simulink model "nms3D_2021"  (R2021a)
settings: Solver=ode15s  StartTime=0.0  StopTime=2  MaxStep=1e-2  RelTol=1e-2
StartFcn:
  | tic
StopFcn:
  | toc
  | 
  | 
  | %if GimbalLockFlag
  |  % fprintf(2, 'Almost reached Gimbal Lock of IMU. Simulation stopped.\n')
  | %end
  | 
  | %fprintf('Elapsed time: %4.2f sec (%4.2f%% realtime)\n', a, tout(end)/a*100)
values from neighbouring files (symbols this model uses):
  Balance02 = pMod(24:29)    [AssignSimulinkParams.m]    (also in assign_parameters.m = param(26:29))
  Balance13 = pMod(30:35)    [AssignSimulinkParams.m]    (also in assign_parameters.m = param(30:33))
  BalanceTrunk = pMod(22:23)    [AssignSimulinkParams.m]    (also in assign_parameters.m = param(22:23))
  BalanceTrunkLat = param(24:25)    [assign_parameters.m]
  BalanceTrunkLatOld = pMod(43:46)    [AssignSimulinkParams.m]    (also in assign_parameters.m = param(43:46))
  BalanceTrunkOld = param(49:53)    [assign_parameters.m]
  BasisStim = pMod(1:11)    [AssignSimulinkParams.m]    (also in assign_parameters.m = param(1:11))
  CompliantLeg = pMod(12:14)    [AssignSimulinkParams.m]    (also in assign_parameters.m = param(12:14))
  CompliantLegLat = pMod(15)    [AssignSimulinkParams.m]    (also in assign_parameters.m = param(15))
  PreventKneeOverextension = pMod(16:21)    [AssignSimulinkParams.m]    (also in assign_parameters.m = param(16:21))
  SwingCompLatOld = param(47:48)    [assign_parameters.m]
  Target02 = pMod(36:38)    [AssignSimulinkParams.m]    (also in assign_parameters.m = param(34:36))
  Target02_va = pMod(49:54)    [AssignSimulinkParams.m]    (also in assign_parameters.m = param(60:65))
  Target13 = pMod(39:41)    [AssignSimulinkParams.m]    (also in assign_parameters.m = param(37:39))
  Target13_va = pMod(55:60)    [AssignSimulinkParams.m]    (also in assign_parameters.m = param(66:71))
  theta0_world = param(59)    [assign_parameters.m]
  WramameiSL_1000 = readmatrix('WSL_1000_Norm_Sigmoid_MSE_cont.csv')    [nms3D_prep.m]
  ZramameiSL_1000 = readmatrix('ZSL_1000_Norm_Sigmoid_MSE_cont.csv')    [nms3D_prep.m]
undefined symbols (not defined in the file or in its folder): ICs, mParams, X, Y, Z
libraries: nesl_utility x106, sm_lib x87, simulink x70, eeGeneralControl x28, robotmaniplib x14, dspinverses x10, robotcorelib x5, dspmathops x3, vrlib x1, pid_lib x1
(part 2 of 8)

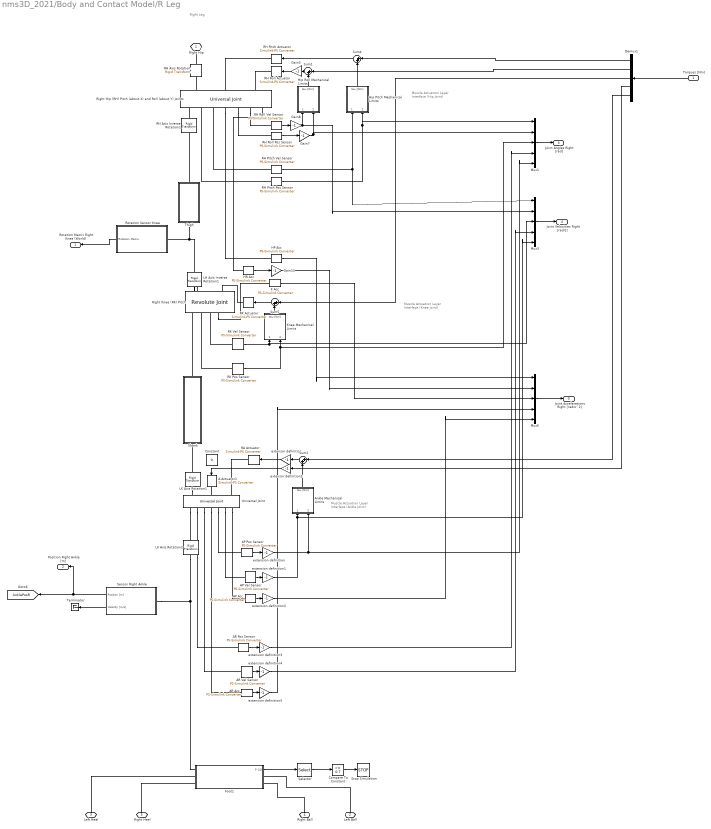
== system nms3D_2021/Body and Contact Model/R Leg ==
  note: Muscle Actuation
      | Layer Interface
      | (Hip Joint)
  note: Muscle Actuation
      | Layer Interface
      | (Knee Joint)
  note: Muscle Actuation
      | Layer Interface
      | (Ankle Joint)
  note: Right Leg
  Torques [Nm] : Inport
  A Actuator1 : nesl_utility/Simulink-PS Converter  PhysicalDomain=network_engine_domain  SubClassName=ps_input  LeftPortType=input  RightPortType=output  PseudoPeriodic=off  Frequencies=[]  NoiseDistribution=none  NoiseParameters=[]  Unit=N*m  AffineConversion=off  FilteringAndDerivatives=zero  SimscapeFilterOrder=1  InputFilterTimeConstant=.001  UdotUserProvided=0
      settings: SourceProductBaseCode=PW,SS
  AP Acc : nesl_utility/PS-Simulink Converter  PhysicalDomain=network_engine_domain  SubClassName=ps_output  LeftPortType=input  RightPortType=output  PseudoPeriodic=off  Frequencies=[]  Unit=rad/(s^2)  AffineConversion=off
      settings: SourceProductBaseCode=PW,SS
  AP Pos Sensor : nesl_utility/PS-Simulink Converter  PhysicalDomain=network_engine_domain  SubClassName=ps_output  LeftPortType=input  RightPortType=output  PseudoPeriodic=off  Frequencies=[]  Unit=rad  AffineConversion=off
      settings: SourceProductBaseCode=PW,SS
  AP Vel Sensor : nesl_utility/PS-Simulink Converter  PhysicalDomain=network_engine_domain  SubClassName=ps_output  LeftPortType=input  RightPortType=output  PseudoPeriodic=off  Frequencies=[]  Unit=rad/s  AffineConversion=off
      settings: SourceProductBaseCode=PW,SS
  AR Acc : nesl_utility/PS-Simulink Converter  PhysicalDomain=network_engine_domain  SubClassName=ps_output  LeftPortType=input  RightPortType=output  PseudoPeriodic=off  Frequencies=[]  Unit=rad/(s^2)  AffineConversion=off
      settings: SourceProductBaseCode=PW,SS
  AR Pos Sensor : nesl_utility/PS-Simulink Converter  PhysicalDomain=network_engine_domain  SubClassName=ps_output  LeftPortType=input  RightPortType=output  PseudoPeriodic=off  Frequencies=[]  Unit=rad  AffineConversion=off
      settings: SourceProductBaseCode=PW,SS
  AR Vel Sensor : nesl_utility/PS-Simulink Converter  PhysicalDomain=network_engine_domain  SubClassName=ps_output  LeftPortType=input  RightPortType=output  PseudoPeriodic=off  Frequencies=[]  Unit=rad/s  AffineConversion=off
      settings: SourceProductBaseCode=PW,SS
  Ankle Mechanical Limits : Subsystem
  Compare To Constant : simulink/Logic and Bit Operations/Compare To Constant  relop=>=  const=0.7  OutDataTypeStr=boolean
  Constant : Constant  Value=0
  Demux1 : Demux  Outputs=5
  Foot1 : Subsystem
  Gain{3,7..8,11} (4 alike) : Gain  Gain=-1
  HP Acc : nesl_utility/PS-Simulink Converter  PhysicalDomain=network_engine_domain  SubClassName=ps_output  LeftPortType=input  RightPortType=output  PseudoPeriodic=off  Frequencies=[]  Unit=rad/(s^2)  AffineConversion=off
      settings: SourceProductBaseCode=PW,SS
  HR Acc : nesl_utility/PS-Simulink Converter  PhysicalDomain=network_engine_domain  SubClassName=ps_output  LeftPortType=input  RightPortType=output  PseudoPeriodic=off  Frequencies=[]  Unit=rad/(s^2)  AffineConversion=off
      settings: SourceProductBaseCode=PW,SS
  Hip Pitch Mechanical Limits : Subsystem
  Hip Roll Mechanical Limits : Subsystem
  K Acc : nesl_utility/PS-Simulink Converter  PhysicalDomain=network_engine_domain  SubClassName=ps_output  LeftPortType=input  RightPortType=output  PseudoPeriodic=off  Frequencies=[]  Unit=rad/(s^2)  AffineConversion=off
      settings: SourceProductBaseCode=PW,SS
  Knee Mechanical Limits : Subsystem
  LH Axis Inverse Rotation1 : sm_lib/Frames and Transforms/Rigid Transform  TranslationMethod=None  TranslationStandardOffset=-0.5  TranslationLengthUnit=m  TranslationStandardAxis=+Y  TranslationCartesianOffset=0  TranslationROffset=0  TranslationROffsetUnits=m  TranslationZOffset=0  TranslationZOffsetUnits=m  TranslationThetaOffset=0  TranslationThetaOffsetUnits=deg  RotationMethod=RotationSequence  RotationAngleUnits=deg  RotationStandardAxis=+X  RotationAngle=-90  RotationArbitraryAxis=[0 0 1]  FollAlignAxisA=+X  BaseAlignAxisA=+Y  FollAlignAxisB=+Y  BaseAlignAxisB=+Z  RotationSequenceAxes=BaseAxes  RotationSequence=ZXZ  RotationSequenceAngles=[180 0 0]  RotationSequenceAnglesUnits=deg  RotationMatrix=[1 0 0; 0 1 0; 0 0 1]
  LK Axis Rotation1 : sm_lib/Frames and Transforms/Rigid Transform  TranslationMethod=None  TranslationStandardOffset=-0.5  TranslationLengthUnit=m  TranslationStandardAxis=+Y  TranslationCartesianOffset=0  TranslationROffset=0  TranslationROffsetUnits=m  TranslationZOffset=0  TranslationZOffsetUnits=m  TranslationThetaOffset=0  TranslationThetaOffsetUnits=deg  RotationMethod=StandardAxis  RotationAngleUnits=deg  RotationStandardAxis=+X  RotationAngle=90  RotationArbitraryAxis=[0 0 1]  FollAlignAxisA=+X  BaseAlignAxisA=+Y  FollAlignAxisB=+Y  BaseAlignAxisB=+Z  RotationSequenceAxes=BaseAxes  RotationSequence=ZXZ  RotationSequenceAngles=[180 0 0]  RotationSequenceAnglesUnits=deg  RotationMatrix=[1 0 0; 0 1 0; 0 0 1]
  LK Axis Rotation2 : sm_lib/Frames and Transforms/Rigid Transform  TranslationMethod=None  TranslationStandardOffset=-0.5  TranslationLengthUnit=m  TranslationStandardAxis=+Y  TranslationCartesianOffset=0  TranslationROffset=0  TranslationROffsetUnits=m  TranslationZOffset=0  TranslationZOffsetUnits=m  TranslationThetaOffset=0  TranslationThetaOffsetUnits=deg  RotationMethod=StandardAxis  RotationAngleUnits=deg  RotationStandardAxis=+X  RotationAngle=-90  RotationArbitraryAxis=[0 0 1]  FollAlignAxisA=+X  BaseAlignAxisA=+Y  FollAlignAxisB=+Y  BaseAlignAxisB=+Z  RotationSequenceAxes=BaseAxes  RotationSequence=ZXZ  RotationSequenceAngles=[180 0 0]  RotationSequenceAnglesUnits=deg  RotationMatrix=[1 0 0; 0 1 0; 0 0 1]
  Mux1 : Mux  Inputs=5
  Mux3 : Mux  Inputs=5
  Mux5 : Mux  Inputs=5
  RA Actuator : nesl_utility/Simulink-PS Converter  PhysicalDomain=network_engine_domain  SubClassName=ps_input  LeftPortType=input  RightPortType=output  PseudoPeriodic=off  Frequencies=[]  NoiseDistribution=none  NoiseParameters=[]  Unit=N*m  AffineConversion=off  FilteringAndDerivatives=zero  SimscapeFilterOrder=1  InputFilterTimeConstant=.001  UdotUserProvided=0
      settings: SourceProductBaseCode=PW,SS
  RH Pitch Pos Sensor : nesl_utility/PS-Simulink Converter  PhysicalDomain=network_engine_domain  SubClassName=ps_output  LeftPortType=input  RightPortType=output  PseudoPeriodic=off  Frequencies=[]  Unit=rad  AffineConversion=off
      settings: SourceProductBaseCode=PW,SS
  RH Pitch Vel Sensor : nesl_utility/PS-Simulink Converter  PhysicalDomain=network_engine_domain  SubClassName=ps_output  LeftPortType=input  RightPortType=output  PseudoPeriodic=off  Frequencies=[]  Unit=rad/s  AffineConversion=off
      settings: SourceProductBaseCode=PW,SS
  RH Roll Pos Sensor : nesl_utility/PS-Simulink Converter  PhysicalDomain=network_engine_domain  SubClassName=ps_output  LeftPortType=input  RightPortType=output  PseudoPeriodic=off  Frequencies=[]  Unit=rad  AffineConversion=off
      settings: SourceProductBaseCode=PW,SS
  "RH Roll Vel Sensor " : nesl_utility/PS-Simulink Converter  PhysicalDomain=network_engine_domain  SubClassName=ps_output  LeftPortType=input  RightPortType=output  PseudoPeriodic=off  Frequencies=[]  Unit=rad/s  AffineConversion=off
      settings: SourceProductBaseCode=PW,SS
  RH Axis Inverse Rotation1 : sm_lib/Frames and Transforms/Rigid Transform  TranslationMethod=None  TranslationStandardOffset=-0.5  TranslationLengthUnit=m  TranslationStandardAxis=+Y  TranslationCartesianOffset=[0 0.2 0]  TranslationROffset=0  TranslationROffsetUnits=m  TranslationZOffset=0  TranslationZOffsetUnits=m  TranslationThetaOffset=0  TranslationThetaOffsetUnits=deg  RotationMethod=RotationSequence  RotationAngleUnits=deg  RotationStandardAxis=+X  RotationAngle=-90  RotationArbitraryAxis=[0 0 1]  FollAlignAxisA=+X  BaseAlignAxisA=+Y  FollAlignAxisB=+Y  BaseAlignAxisB=+Z  RotationSequenceAxes=BaseAxes  RotationSequence=YXY  RotationSequenceAngles=[ -90 -90 0]  RotationSequenceAnglesUnits=deg  RotationMatrix=[1 0 0; 0 1 0; 0 0 1]
  RH Axis Rotation : sm_lib/Frames and Transforms/Rigid Transform  TranslationMethod=None  TranslationStandardOffset=-0  TranslationLengthUnit=m  TranslationStandardAxis=+Y  TranslationCartesianOffset=0  TranslationROffset=0  TranslationROffsetUnits=m  TranslationZOffset=0  TranslationZOffsetUnits=m  TranslationThetaOffset=0  TranslationThetaOffsetUnits=deg  RotationMethod=RotationSequence  RotationAngleUnits=deg  RotationStandardAxis=+X  RotationAngle=90  RotationArbitraryAxis=[0 0 1]  FollAlignAxisA=+X  BaseAlignAxisA=+Y  FollAlignAxisB=+Y  BaseAlignAxisB=+Z  RotationSequenceAxes=FollowerAxes  RotationSequence=XZX  RotationSequenceAngles=[-90 90 0]  RotationSequenceAnglesUnits=deg  RotationMatrix=[1 0 0; 0 1 0; 0 0 1]
  RH Pitch Actuator : nesl_utility/Simulink-PS Converter  PhysicalDomain=network_engine_domain  SubClassName=ps_input  LeftPortType=input  RightPortType=output  PseudoPeriodic=off  Frequencies=[]  NoiseDistribution=none  NoiseParameters=[]  Unit=N*m  AffineConversion=off  FilteringAndDerivatives=zero  SimscapeFilterOrder=1  InputFilterTimeConstant=.001  UdotUserProvided=0
      settings: SourceProductBaseCode=PW,SS
  RH Roll Actuator : nesl_utility/Simulink-PS Converter  PhysicalDomain=network_engine_domain  SubClassName=ps_input  LeftPortType=input  RightPortType=output  PseudoPeriodic=off  Frequencies=[]  NoiseDistribution=none  NoiseParameters=[]  Unit=N*m  AffineConversion=off  FilteringAndDerivatives=zero  SimscapeFilterOrder=1  InputFilterTimeConstant=.001  UdotUserProvided=0
      settings: SourceProductBaseCode=PW,SS
  RK Actuator : nesl_utility/Simulink-PS Converter  PhysicalDomain=network_engine_domain  SubClassName=ps_input  LeftPortType=input  RightPortType=output  PseudoPeriodic=off  Frequencies=[]  NoiseDistribution=none  NoiseParameters=[]  Unit=N*m  AffineConversion=off  FilteringAndDerivatives=zero  SimscapeFilterOrder=1  InputFilterTimeConstant=.001  UdotUserProvided=0
      settings: SourceProductBaseCode=PW,SS
  RK Pos Sensor : nesl_utility/PS-Simulink Converter  PhysicalDomain=network_engine_domain  SubClassName=ps_output  LeftPortType=input  RightPortType=output  PseudoPeriodic=off  Frequencies=[]  Unit=rad  AffineConversion=off
      settings: SourceProductBaseCode=PW,SS
  RK Vel Sensor : nesl_utility/PS-Simulink Converter  PhysicalDomain=network_engine_domain  SubClassName=ps_output  LeftPortType=input  RightPortType=output  PseudoPeriodic=off  Frequencies=[]  Unit=rad/s  AffineConversion=off
      settings: SourceProductBaseCode=PW,SS
  Right Hip (RH) Pitch (about X) and Roll (about Y) Joints : sm_lib/Joints/Universal Joint  JointMode=Normal  SenseConstraintForce=off  SenseConstraintForceX=off  SenseConstraintForceY=off  SenseConstraintForceZ=off  SenseConstraintTorque=off  SenseConstraintTorqueX=off  SenseConstraintTorqueY=off  SenseConstraintTorqueZ=off  SenseTotalForce=off  SenseTotalForceX=off  SenseTotalForceY=off  SenseTotalForceZ=off  SenseTotalTorque=off  SenseTotalTorqueX=off  SenseTotalTorqueY=off  SenseTotalTorqueZ=off  CompositeWrenchDir=FollowerOnBase  CompositeWrenchFrame=FollowerFrame  RxEquilibriumPosition=0  RxEquilibriumPositionUnits=deg  RxSpringStiffness=0  RxSpringStiffnessUnits=N*m/deg  RxDampingCoefficient=0  RxDampingCoefficientUnits=N*m/(deg/s)  RxTorqueActuationMode=InputTorque  RxMotionActuationMode=ComputedMotion  RxSensePosition=on  RxSenseVelocity=on  RxSenseAcceleration=on  RxSenseTorqueForce=off  RxSenseLowerLimitTorqueForce=off  RxSenseUpperLimitTorqueForce=off  RxLowerLimitSpecify=off  RxLowerLimitBound=-90  RxLowerLimitBoundUnits=deg  RxLowerLimitStiffness=1e4  RxLowerLimitStiffnessUnits=N*m/deg  RxLowerLimitDamping=10  RxLowerLimitDampingUnits=N*m/(deg/s)  RxLowerLimitTransitionRegionWidth=0.1  RxLowerLimitTransitionRegionWidthUnits=deg  RxUpperLimitSpecify=off  RxUpperLimitBound=90  RxUpperLimitBoundUnits=deg  RxUpperLimitStiffness=1e4  RxUpperLimitStiffnessUnits=N*m/deg  RxUpperLimitDamping=10  RxUpperLimitDampingUnits=N*m/(deg/s)  RxUpperLimitTransitionRegionWidth=0.1  RxUpperLimitTransitionRegionWidthUnits=deg  RxPositionTargetSpecify=on  RxPositionTargetPriority=High  RxPositionTargetValue=ICs.rLeg.hip.qP0  RxPositionTargetValueUnits=rad  RxVelocityTargetSpecify=on  RxVelocityTargetPriority=High  RxVelocityTargetValue=0  RxVelocityTargetValueUnits=rad/s  RyEquilibriumPosition=0  RyEquilibriumPositionUnits=deg  RySpringStiffness=0  RySpringStiffnessUnits=N*m/deg  RyDampingCoefficient=0  RyDampingCoefficientUnits=N*m/(deg/s)  RyTorqueActuationMode=InputTorque  RyMotionActuationMode=ComputedMotion  RySensePosition=on  RySenseVelocity=on  RySenseAcceleration=on  RySenseTorqueForce=off  RySenseLowerLimitTorqueForce=off  RySenseUpperLimitTorqueForce=off  RyLowerLimitSpecify=off  RyLowerLimitBound=-90  RyLowerLimitBoundUnits=deg  RyLowerLimitStiffness=1e4  RyLowerLimitStiffnessUnits=N*m/deg  RyLowerLimitDamping=10  RyLowerLimitDampingUnits=N*m/(deg/s)  RyLowerLimitTransitionRegionWidth=0.1  RyLowerLimitTransitionRegionWidthUnits=deg  RyUpperLimitSpecify=off  RyUpperLimitBound=90  RyUpperLimitBoundUnits=deg  RyUpperLimitStiffness=1e4  RyUpperLimitStiffnessUnits=N*m/deg  RyUpperLimitDamping=10  RyUpperLimitDampingUnits=N*m/(deg/s)  RyUpperLimitTransitionRegionWidth=0.1  RyUpperLimitTransitionRegionWidthUnits=deg  RyPositionTargetSpecify=on  RyPositionTargetPriority=High  RyPositionTargetValue=-ICs.rLeg.hip.qR0  RyPositionTargetValueUnits=rad  RyVelocityTargetSpecify=on  RyVelocityTargetPriority=High  RyVelocityTargetValue=0  RyVelocityTargetValueUnits=rad/s
  Right Knee (RK) Pitch : sm_lib/Joints/Revolute Joint  JointMode=Normal  SenseConstraintForce=off  SenseConstraintForceX=off  SenseConstraintForceY=off  SenseConstraintForceZ=off  SenseConstraintTorque=off  SenseConstraintTorqueX=off  SenseConstraintTorqueY=off  SenseConstraintTorqueZ=off  SenseTotalForce=off  SenseTotalForceX=off  SenseTotalForceY=off  SenseTotalForceZ=off  SenseTotalTorque=off  SenseTotalTorqueX=off  SenseTotalTorqueY=off  SenseTotalTorqueZ=off  CompositeWrenchDir=FollowerOnBase  CompositeWrenchFrame=FollowerFrame  EquilibriumPosition=0  EquilibriumPositionUnits=deg  SpringStiffness=0  SpringStiffnessUnits=N*m/deg  DampingCoefficient=0  DampingCoefficientUnits=N*m/(deg/s)  TorqueActuationMode=InputTorque  MotionActuationMode=ComputedMotion  SensePosition=on  SenseVelocity=on  SenseAcceleration=on  SenseTorqueForce=on  SenseLowerLimitTorqueForce=off  SenseUpperLimitTorqueForce=off  LowerLimitSpecify=off  LowerLimitBound=-90  LowerLimitBoundUnits=deg  LowerLimitStiffness=1e4  LowerLimitStiffnessUnits=N*m/deg  LowerLimitDamping=10  LowerLimitDampingUnits=N*m/(deg/s)  LowerLimitTransitionRegionWidth=0.1  LowerLimitTransitionRegionWidthUnits=deg  UpperLimitSpecify=off  UpperLimitBound=90  UpperLimitBoundUnits=deg  UpperLimitStiffness=1e4  UpperLimitStiffnessUnits=N*m/deg  UpperLimitDamping=10  UpperLimitDampingUnits=N*m/(deg/s)  UpperLimitTransitionRegionWidth=0.1  UpperLimitTransitionRegionWidthUnits=deg  PositionTargetSpecify=on  PositionTargetPriority=High  PositionTargetValue=ICs.rLeg.knee.qP0  PositionTargetValueUnits=rad  VelocityTargetSpecify=on  VelocityTargetPriority=High  VelocityTargetValue=0  VelocityTargetValueUnits=rad/s
  Rotation Sensor Knee : Subsystem
  Selector : Selector  InputPortWidth=3  IndexOptions=Index vector (dialog)  Indices=[2]  OutputSizes=1
  Sensor Right Ankle : Subsystem
  Shank : Subsystem
  Stop Simulation : Stop
  Sum{1..2,4..5} (4 alike) : Sum  Inputs=|++
  Terminator : Terminator
  Thigh : Subsystem
  Universal Joint : sm_lib/Joints/Universal Joint  JointMode=Normal  SenseConstraintForce=off  SenseConstraintForceX=off  SenseConstraintForceY=off  SenseConstraintForceZ=off  SenseConstraintTorque=off  SenseConstraintTorqueX=off  SenseConstraintTorqueY=off  SenseConstraintTorqueZ=off  SenseTotalForce=off  SenseTotalForceX=off  SenseTotalForceY=off  SenseTotalForceZ=off  SenseTotalTorque=off  SenseTotalTorqueX=off  SenseTotalTorqueY=off  SenseTotalTorqueZ=off  CompositeWrenchDir=FollowerOnBase  CompositeWrenchFrame=BaseFrame  RxEquilibriumPosition=0  RxEquilibriumPositionUnits=deg  RxSpringStiffness=0  RxSpringStiffnessUnits=N*m/deg  RxDampingCoefficient=0  RxDampingCoefficientUnits=N*m/(deg/s)  RxTorqueActuationMode=InputTorque  RxMotionActuationMode=ComputedMotion  RxSensePosition=on  RxSenseVelocity=on  RxSenseAcceleration=on  RxSenseTorqueForce=off  RxSenseLowerLimitTorqueForce=off  RxSenseUpperLimitTorqueForce=off  RxLowerLimitSpecify=off  RxLowerLimitBound=-90  RxLowerLimitBoundUnits=deg  RxLowerLimitStiffness=1e4  RxLowerLimitStiffnessUnits=N*m/deg  RxLowerLimitDamping=10  RxLowerLimitDampingUnits=N*m/(deg/s)  RxLowerLimitTransitionRegionWidth=0.1  RxLowerLimitTransitionRegionWidthUnits=deg  RxUpperLimitSpecify=off  RxUpperLimitBound=90  RxUpperLimitBoundUnits=deg  RxUpperLimitStiffness=1e4  RxUpperLimitStiffnessUnits=N*m/deg  RxUpperLimitDamping=10  RxUpperLimitDampingUnits=N*m/(deg/s)  RxUpperLimitTransitionRegionWidth=0.1  RxUpperLimitTransitionRegionWidthUnits=deg  RxPositionTargetSpecify=on  RxPositionTargetPriority=High  RxPositionTargetValue=0  RxPositionTargetValueUnits=rad  RxVelocityTargetSpecify=on  RxVelocityTargetPriority=High  RxVelocityTargetValue=0  RxVelocityTargetValueUnits=deg/s  RyEquilibriumPosition=0  RyEquilibriumPositionUnits=deg  RySpringStiffness=0  RySpringStiffnessUnits=N*m/deg  RyDampingCoefficient=0  RyDampingCoefficientUnits=N*m/(deg/s)  RyTorqueActuationMode=InputTorque  RyMotionActuationMode=ComputedMotion  RySensePosition=on  RySenseVelocity=on  RySenseAcceleration=on  RySenseTorqueForce=off  RySenseLowerLimitTorqueForce=off  RySenseUpperLimitTorqueForce=off  RyLowerLimitSpecify=off  RyLowerLimitBound=-90  RyLowerLimitBoundUnits=deg  RyLowerLimitStiffness=1e4  RyLowerLimitStiffnessUnits=N*m/deg  RyLowerLimitDamping=10  RyLowerLimitDampingUnits=N*m/(deg/s)  RyLowerLimitTransitionRegionWidth=0.1  RyLowerLimitTransitionRegionWidthUnits=deg  RyUpperLimitSpecify=off  RyUpperLimitBound=90  RyUpperLimitBoundUnits=deg  RyUpperLimitStiffness=1e4  RyUpperLimitStiffnessUnits=N*m/deg  RyUpperLimitDamping=10  RyUpperLimitDampingUnits=N*m/(deg/s)  RyUpperLimitTransitionRegionWidth=0.1  RyUpperLimitTransitionRegionWidthUnits=deg  RyPositionTargetSpecify=on  RyPositionTargetPriority=High  RyPositionTargetValue=-ICs.rLeg.ankle.qP0  RyPositionTargetValueUnits=rad  RyVelocityTargetSpecify=off  RyVelocityTargetPriority=High  RyVelocityTargetValue=0  RyVelocityTargetValueUnits=deg/s
  extension definition{,1..5} (6 alike) : Gain  Gain=-1
  extensor definition : Gain  Gain=-1
  extensor definition1 : Gain  Gain=-1
  Right Hip : PMIOPort  Side=Left
  "Left Ball " : PMIOPort  Port=2  Side=Right
  Left Heel : PMIOPort  Port=3  Side=Right
  Right Ball : PMIOPort  Port=4  Side=Right
  Right Heel : PMIOPort  Port=5  Side=Right
  Rotation Matrix Right Knee (World) : Outport
  Position Right Ankle [m] : Outport  Port=2
  Joint Angles Right [rad] : Outport  Port=3
  "Joint Velocities Right [rad/s] " : Outport  Port=4
  Joint Accelerations Right [rad/s^2] : Outport  Port=5
  tag scope: AnklePosR=global
  wires:
  Hip Pitch Mechanical Limits/1(tau [Nm]) -> Sum4/2
  RH Pitch Vel Sensor/1 -> Mux3/1, Hip Pitch Mechanical Limits/1(dq [rad/s])
  Hip Roll Mechanical Limits/1(tau [Nm]) -> Sum1/2
  RK Pos Sensor/1 -> Knee Mechanical Limits/2(q [rad]), Mux1/3
  Demux1/3 -> Sum5/1
  RK Vel Sensor/1 -> Mux3/3, Knee Mechanical Limits/1(dq [rad/s])
  RH Pitch Pos Sensor/1 -> Hip Pitch Mechanical Limits/2(q [rad]), Mux1/1
  RH Roll Pos Sensor/1 -> Gain7/1
  Demux1/1 -> Sum4/1
  Sum2/1 -> extensor definition/1
  AP Vel Sensor/1 -> extension definition1/1
  Ankle Mechanical Limits/1(tau [Nm]) -> Sum2/2
  AP Pos Sensor/1 -> extension definition/1
  extension definition/1 -> Ankle Mechanical Limits/2(q [rad]), Mux1/5
  extension definition1/1 -> Mux3/5, Ankle Mechanical Limits/1(dq [rad/s])
  Sum4/1 -> RH Pitch Actuator/1
  Sum1/1 -> Gain3/1
  Gain3/1 -> RH Roll Actuator/1
  Sum5/1 -> RK Actuator/1
  extensor definition/1 -> RA Actuator/1
  "RH Roll Vel Sensor "/1 -> Gain8/1
  Gain8/1 -> Mux3/2, Hip Roll Mechanical Limits/1(dq [rad/s])
  Gain7/1 -> Mux1/2, Hip Roll Mechanical Limits/2(q [rad])
  Demux1/2 -> Sum1/1
  Mux3/1 -> "Joint Velocities Right [rad/s] "/1
  Mux5/1 -> Joint Accelerations Right [rad/s^2]/1
  HP Acc/1 -> Mux5/1
  HR Acc/1 -> Gain11/1
  Gain11/1 -> Mux5/2
  K Acc/1 -> Mux5/3
  AP Acc/1 -> extension definition2/1
  extension definition2/1 -> Mux5/5
  Knee Mechanical Limits/1(tau [Nm]) -> Sum5/2
  Sensor Right Ankle/1(Position [m]) -> Position Right Ankle [m]/1, [AnklePosR]
  Rotation Sensor Knee/1(Rotation Matrix) -> Rotation Matrix Right Knee (World)/1
  Selector/1 -> Compare To Constant/1
  Compare To Constant/1 -> Stop Simulation/1
  Foot1/1(P CG) -> Selector/1
  Sensor Right Ankle/2(Velocity [m/s]) -> Terminator/1
  Torques [Nm]/1 -> Demux1/1
  Mux1/1 -> Joint Angles Right [rad]/1
  AR Pos Sensor/1 -> extension definition3/1
  AR Vel Sensor/1 -> extension definition4/1
  AR Acc/1 -> extension definition5/1
  extension definition3/1 -> Mux1/4
  extension definition4/1 -> Mux3/4
  extension definition5/1 -> Mux5/4
  Demux1/5 -> Sum2/1
  Demux1/4 -> extensor definition1/1
  extensor definition1/1 -> A Actuator1/1
  connections:
  RH Axis Rotation/LConn1 -- Right Hip/RConn1
  RK Vel Sensor/LConn1 -- Right Knee (RK) Pitch/RConn3
  RK Pos Sensor/LConn1 -- Right Knee (RK) Pitch/RConn2
  RH Pitch Pos Sensor/LConn1 -- Right Hip (RH) Pitch (about X) and Roll (about Y) Joints/RConn2
  RH Pitch Vel Sensor/LConn1 -- Right Hip (RH) Pitch (about X) and Roll (about Y) Joints/RConn3
  Right Hip (RH) Pitch (about X) and Roll (about Y) Joints/LConn1 -- RH Axis Rotation/RConn1
  Shank/LConn1 -- Right Knee (RK) Pitch/RConn1
  LH Axis Inverse Rotation1/RConn1 -- Right Knee (RK) Pitch/LConn1
  LK Axis Rotation1/LConn1 -- Shank/RConn1
  RH Axis Inverse Rotation1/LConn1 -- Right Hip (RH) Pitch (about X) and Roll (about Y) Joints/RConn1
  Right Hip (RH) Pitch (about X) and Roll (about Y) Joints/RConn5 -- RH Roll Pos Sensor/LConn1
  Right Hip (RH) Pitch (about X) and Roll (about Y) Joints/RConn6 -- "RH Roll Vel Sensor "/LConn1
  Right Hip (RH) Pitch (about X) and Roll (about Y) Joints/RConn4 -- HP Acc/LConn1
  Right Hip (RH) Pitch (about X) and Roll (about Y) Joints/RConn7 -- HR Acc/LConn1
  Right Knee (RK) Pitch/RConn4 -- K Acc/LConn1
  Right Heel/RConn1 -- Foot1/LConn3
  Left Heel/RConn1 -- Foot1/LConn2
  Right Ball/RConn1 -- Foot1/RConn2
  "Left Ball "/RConn1 -- Foot1/RConn1
  Thigh/LConn1 -- RH Axis Inverse Rotation1/RConn1
  Thigh/RConn1 -- LH Axis Inverse Rotation1/LConn1 -- Rotation Sensor Knee/LConn1
  Sensor Right Ankle/LConn1 -- LK Axis Rotation2/RConn1 -- Foot1/LConn1
  RK Actuator/RConn1 -- Right Knee (RK) Pitch/LConn2
  RH Pitch Actuator/RConn1 -- Right Hip (RH) Pitch (about X) and Roll (about Y) Joints/LConn2
  RH Roll Actuator/RConn1 -- Right Hip (RH) Pitch (about X) and Roll (about Y) Joints/LConn3
  RA Actuator/RConn1 -- Universal Joint/LConn3
  Universal Joint/RConn6 -- AP Vel Sensor/LConn1
  Universal Joint/RConn5 -- AP Pos Sensor/LConn1
  Universal Joint/RConn7 -- AP Acc/LConn1
  LK Axis Rotation1/RConn1 -- Universal Joint/LConn1
  Universal Joint/RConn1 -- LK Axis Rotation2/LConn1
  Universal Joint/RConn2 -- AR Pos Sensor/LConn1
  Universal Joint/RConn3 -- AR Vel Sensor/LConn1
  Universal Joint/RConn4 -- AR Acc/LConn1
  Universal Joint/LConn2 -- A Actuator1/RConn1

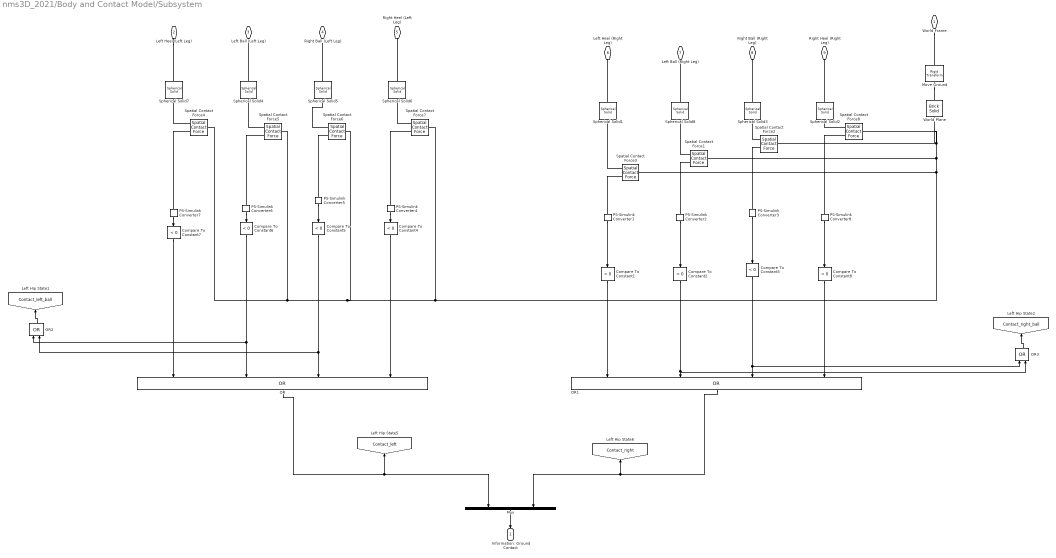
== system nms3D_2021/Body and Contact Model/Subsystem ==
  Compare To Constant{1..8} (8 alike) : simulink/Logic and Bit Operations/Compare To Constant  relop=<  const=0  OutDataTypeStr=boolean
  Move Ground : sm_lib/Frames and Transforms/Rigid Transform  TranslationMethod=StandardAxis  TranslationStandardOffset=-0.05  TranslationLengthUnit=m  TranslationStandardAxis=+Y  TranslationCartesianOffset=0  TranslationROffset=0  TranslationROffsetUnits=m  TranslationZOffset=0  TranslationZOffsetUnits=m  TranslationThetaOffset=0  TranslationThetaOffsetUnits=deg  RotationMethod=None  RotationAngleUnits=deg  RotationStandardAxis=+X  RotationAngle=-90  RotationArbitraryAxis=[0 0 1]  FollAlignAxisA=+X  BaseAlignAxisA=+Y  FollAlignAxisB=+Y  BaseAlignAxisB=+Z  RotationSequenceAxes=BaseAxes  RotationSequence=ZXZ  RotationSequenceAngles=[180 0 0]  RotationSequenceAnglesUnits=deg  RotationMatrix=[1 0 0; 0 1 0; 0 0 1]
  Mux : Mux  Inputs=2
  OR : Logic  Operator=OR  Inputs=4  AllPortsSameDT=off  OutDataTypeStr=boolean
  OR1 : Logic  Operator=OR  Inputs=4  AllPortsSameDT=off  OutDataTypeStr=boolean
  OR2 : Logic  Operator=OR  AllPortsSameDT=off  OutDataTypeStr=boolean
  OR3 : Logic  Operator=OR  AllPortsSameDT=off  OutDataTypeStr=boolean
  PS-Simulink Converter{1..8} (8 alike) : nesl_utility/PS-Simulink Converter  PhysicalDomain=network_engine_domain  SubClassName=ps_output  LeftPortType=input  RightPortType=output  PseudoPeriodic=off  Frequencies=[]  Unit=m  AffineConversion=off
      settings: SourceProductBaseCode=PW,SS
  Spatial Contact Force{1..8} (8 alike) : sm_lib/Forces and Torques/Spatial Contact Force  CoefficientOfDynamicFriction=mParams.Contacts.mu_k  CoefficientOfStaticFriction=mParams.Contacts.mu_s  SenseContactBaseRotation=off  SenseContactBaseTranslation=off  NormalDamping=mParams.Contacts.damping  NormalDampingUnits=N/(m/s)  SenseContactFollowerRotation=off  SenseContactFollowerTranslation=off  SenseContactSignal=off  NormalStiffness=mParams.Contacts.stiffness  NormalStiffnessUnits=N/m  FrictionalCriticalVelocity=mParams.Contacts.vLimit  FrictionalCriticalVelocityUnits=m/s  ZeroCrossDetectContactStartAndEnd=off  FrictionType=SmoothStickSlip  SenseFrictionalForceMagnitude=off  SenseNormalForceMagnitude=off  NormalForceType=SmoothSpringDamper  SenseNormalVelocity=off  SenseSeparationDistance=on  SenseTangentialVelocity=off  SenseTangentialVelocityMagnitude=off  NormalTransitionRegionWidth=mParams.Contacts.depths  NormalTransitionRegionWidthUnits=m
  Spherical Solid{1..8} (8 alike) : sm_lib/Body Elements/Spherical Solid  GraphicAmbientColor=[0.15 0.15 0.15 1.0]  BasedOnType=Mass  CenterOfMass=[0 0 0]  CenterOfMassUnits=m  GraphicDiffuseColor=[0.5 0.5 0.5]  Density=1000  DensityUnits=kg/m^3  DoExposeReferenceFrame=on  GraphicEmissiveColor=[0.0 0.0 0.0 1.0]  ExportEntireGeometry=on  SerializedExposedGeometries=<ExposedGeometries><ExposedGeometry><RawGeometryId>entire</RawGeometryId><ExposedGeometryId>G</ExposedGeometryId></ExposedGeometry></ExposedGeometries>  SerializedFrames=<Frames/>  MarkerShape=Sphere  MarkerSize=10  GraphicType=FromGeometry  InertiaType=CalculateFromGeometry  Mass=1  MassUnits=g  MomentsOfInertia=[1 1 1]  MomentsOfInertiaUnits=kg*m^2  GraphicOpacity=1.0  ProductsOfInertia=[0 0 0]  ProductsOfInertiaUnits=kg*m^2  GraphicShininess=75  GraphicSpecularColor=[0.5 0.5 0.5 1.0]  SphereRadius=mParams.Contacts.size  SphereRadiusUnits=m  GraphicVisPropType=SimpleVisualProperties
  World Plane : sm_lib/Body Elements/Brick Solid  GraphicAmbientColor=[0.15 0.15 0.15 1.0]  BasedOnType=Density  BrickDimensions=[400 0.1 100]  BrickDimensionUnits=m  CenterOfMass=[0 0 0]  CenterOfMassUnits=m  GraphicDiffuseColor=[1.0 1.0 0.8]  Density=1000  DensityUnits=kg/(m^3)  DoExposeReferenceFrame=on  GraphicEmissiveColor=[0.0 0.0 0.0 1.0]  ExportEntireGeometry=on  SerializedFrames=<Frames/>  MarkerShape=Sphere  MarkerSize=10  GraphicType=FromGeometry  InertiaType=CalculateFromGeometry  Mass=1  MassUnits=kg  MomentsOfInertia=[1 1 1]  MomentsOfInertiaUnits=kg*m^2  GraphicOpacity=0.5  ProductsOfInertia=[0 0 0]  ProductsOfInertiaUnits=kg*m^2  GraphicShininess=75  GraphicSpecularColor=[0.5 0.5 0.5 1.0]  GraphicVisPropType=SimpleVisualProperties
  World Frame : PMIOPort  Side=Left
  Left Heel (Left Leg) : PMIOPort  Port=2  Side=Right
  Left Ball (Left Leg) : PMIOPort  Port=3  Side=Right
  Right Ball (Left Leg) : PMIOPort  Port=4  Side=Right
  Right Heel (Left Leg) : PMIOPort  Port=5  Side=Right
  Left Heel (Right Leg) : PMIOPort  Port=6  Side=Right
  Left Ball (Right Leg) : PMIOPort  Port=7  Side=Right
  Right Ball (Right Leg) : PMIOPort  Port=8  Side=Right
  Right Heel (Right Leg) : PMIOPort  Port=9  Side=Right
  Information: Ground Contact : Outport
  tag scope: Contact_left=global, Contact_left_ball=global, Contact_right=global, Contact_right_ball=global
  wires:
  Compare To Constant1/1 -> OR1/1
  PS-Simulink Converter4/1 -> Compare To Constant4/1
  PS-Simulink Converter5/1 -> Compare To Constant5/1
  Compare To Constant4/1 -> OR/4
  PS-Simulink Converter3/1 -> Compare To Constant3/1
  Compare To Constant6/1 -> OR2/1, OR/2
  PS-Simulink Converter1/1 -> Compare To Constant1/1
  PS-Simulink Converter8/1 -> Compare To Constant8/1
  Compare To Constant3/1 -> OR3/1, OR1/3
  Compare To Constant8/1 -> OR1/4
  PS-Simulink Converter6/1 -> Compare To Constant6/1
  PS-Simulink Converter7/1 -> Compare To Constant7/1
  Compare To Constant2/1 -> OR3/2, OR1/2
  Compare To Constant5/1 -> OR2/2, OR/3
  Compare To Constant7/1 -> OR/1
  PS-Simulink Converter2/1 -> Compare To Constant2/1
  OR1/1 -> [Contact_right], Mux/2
  Mux/1 -> Information: Ground Contact/1
  OR/1 -> Mux/1, [Contact_left]
  OR2/1 -> [Contact_left_ball]
  OR3/1 -> [Contact_right_ball]
  connections:
  Spatial Contact Force7/RConn1 -- Spherical Solid6/LConn1
  Spatial Contact Force5/RConn2 -- PS-Simulink Converter6/LConn1
  Spatial Contact Force1/RConn2 -- PS-Simulink Converter2/LConn1
  Spatial Contact Force7/RConn2 -- PS-Simulink Converter4/LConn1
  Spherical Solid5/RConn1 -- Right Ball (Left Leg)/RConn1
  Spatial Contact Force1/RConn1 -- Spherical Solid8/LConn1
  Spatial Contact Force2/RConn2 -- PS-Simulink Converter3/LConn1
  Spatial Contact Force8/RConn2 -- PS-Simulink Converter8/LConn1
  Spatial Contact Force6/RConn1 -- Spherical Solid5/LConn1
  Spatial Contact Force3/RConn2 -- PS-Simulink Converter1/LConn1
  Spatial Contact Force8/LConn1 -- World Plane/LConn1 -- Spatial Contact Force2/LConn1 -- Spatial Contact Force1/LConn1 -- Spatial Contact Force3/LConn1 -- Spatial Contact Force7/LConn1 -- Spatial Contact Force6/LConn1 -- Spatial Contact Force4/LConn1 -- Spatial Contact Force5/LConn1
  Spatial Contact Force5/RConn1 -- Spherical Solid4/LConn1
  Spatial Contact Force6/RConn2 -- PS-Simulink Converter5/LConn1
  Spatial Contact Force2/RConn1 -- Spherical Solid3/LConn1
  Move Ground/RConn1 -- World Plane/RConn1
  World Frame/RConn1 -- Move Ground/LConn1
  Spatial Contact Force3/RConn1 -- Spherical Solid1/LConn1
  Spherical Solid6/RConn1 -- Right Heel (Left Leg)/RConn1
  Spatial Contact Force4/RConn2 -- PS-Simulink Converter7/LConn1
  Spatial Contact Force4/RConn1 -- Spherical Solid7/LConn1
  Spherical Solid4/RConn1 -- Left Ball (Left Leg)/RConn1
  Spatial Contact Force8/RConn1 -- Spherical Solid2/LConn1
  Left Heel (Left Leg)/RConn1 -- Spherical Solid7/RConn1
  Spherical Solid2/RConn1 -- Right Heel (Right Leg)/RConn1
  Spherical Solid1/RConn1 -- Left Heel (Right Leg)/RConn1
  Spherical Solid3/RConn1 -- Right Ball (Right Leg)/RConn1
  Spherical Solid8/RConn1 -- Left Ball (Right Leg)/RConn1

== system nms3D_2021/Body and Contact Model/Trunk (floating base) ==
  Solid : sm_lib/Body Elements/Brick Solid  GraphicAmbientColor=[0.15 0.15 0.15 1.0]  BasedOnType=Density  BrickDimensions=[mParams.bodies.trunk.d mParams.bodies.trunk.l mParams.bodies.trunk.b]  BrickDimensionUnits=m  CenterOfMass=mParams.bodies.trunk.CG  CenterOfMassUnits=m  GraphicDiffuseColor=[0.5 1 0.5]  Density=2.7  DensityUnits=g/cm^3  DoExposeReferenceFrame=on  GraphicEmissiveColor=[0 0 0 1.0]  ExportEntireGeometry=off  SerializedFrames=<Frames><Frame><Id>Frame1</Id><Value><Name>CG</Name><Origin><Source>CenterOfMassFrame</Source><FeatureName></FeatureName></Origin><PrimaryAxis><DefinedDirection>+Z</DefinedDirection><Source>ReferenceFrame</Source><SourceDirection>+Z</SourceDirection><FeatureName></FeatureName></PrimaryAxis><SecondaryAxis><DefinedDirection>+X</DefinedDirection><Source>ReferenceFrame</Source><SourceDirection>+X</SourceDirection><FeatureName></FeatureName></SecondaryAxis></Value></Frame></Frames>  MarkerShape=Cube  MarkerSize=100  GraphicType=FromGeometry  InertiaType=Custom  Mass=mParams.bodies.trunk.m  MassUnits=kg  MomentsOfInertia=mParams.bodies.trunk.In  MomentsOfInertiaUnits=kg*m^2  GraphicOpacity=0.5  ProductsOfInertia=[0 0 0]  ProductsOfInertiaUnits=kg*m^2  GraphicShininess=75  GraphicSpecularColor=[0.5 0.5 0.5 1.0]  GraphicVisPropType=SimpleVisualProperties
  Transform CG to LH : sm_lib/Frames and Transforms/Rigid Transform  TranslationMethod=Cartesian  TranslationStandardOffset=0  TranslationLengthUnit=m  TranslationStandardAxis=+Y  TranslationCartesianOffset=mParams.bodies.trunk.CG_LH  TranslationROffset=0  TranslationROffsetUnits=m  TranslationZOffset=0  TranslationZOffsetUnits=m  TranslationThetaOffset=0  TranslationThetaOffsetUnits=deg  RotationMethod=None  RotationAngleUnits=deg  RotationStandardAxis=+X  RotationAngle=90  RotationArbitraryAxis=[0 0 1]  FollAlignAxisA=+X  BaseAlignAxisA=+Y  FollAlignAxisB=+Y  BaseAlignAxisB=+Z  RotationSequenceAxes=FollowerAxes  RotationSequence=XYX  RotationSequenceAngles=[0 0 0]  RotationSequenceAnglesUnits=deg  RotationMatrix=[1 0 0; 0 1 0; 0 0 1]
  Transform CG to RH : sm_lib/Frames and Transforms/Rigid Transform  TranslationMethod=Cartesian  TranslationStandardOffset=-0  TranslationLengthUnit=m  TranslationStandardAxis=+Y  TranslationCartesianOffset=mParams.bodies.trunk.CG_RH  TranslationROffset=0  TranslationROffsetUnits=m  TranslationZOffset=0  TranslationZOffsetUnits=m  TranslationThetaOffset=0  TranslationThetaOffsetUnits=deg  RotationMethod=None  RotationAngleUnits=deg  RotationStandardAxis=+X  RotationAngle=90  RotationArbitraryAxis=[0 0 1]  FollAlignAxisA=+X  BaseAlignAxisA=+Y  FollAlignAxisB=+Y  BaseAlignAxisB=+Z  RotationSequenceAxes=FollowerAxes  RotationSequence=XYX  RotationSequenceAngles=[0 0 0]  RotationSequenceAnglesUnits=deg  RotationMatrix=[1 0 0; 0 1 0; 0 0 1]
  CG : PMIOPort  Side=Left
  Left Hip : PMIOPort  Port=2  Side=Right
  Right Hip : PMIOPort  Port=3  Side=Right
  connections:
  Solid/LConn1 -- Transform CG to RH/LConn1 -- Transform CG to LH/LConn1 -- CG/RConn1
  Left Hip/RConn1 -- Transform CG to LH/RConn1
  Right Hip/RConn1 -- Transform CG to RH/RConn1

== system nms3D_2021/Body and Contact Model/Vestibular System ==
  Ankle Position Right [m] : Inport
  Ankle Position Left [m] : Inport  Port=2
  "  XYZ Sensor Left Hip" : Subsystem
  "  XYZ Sensor Right Hip" : Subsystem
  Align Axis : Subsystem
  Compare To Constant : simulink/Logic and Bit Operations/Compare To Constant  relop=<=  const=1  OutDataTypeStr=boolean
  Mux : Mux  Inputs=7
  R Movement direction : Subsystem
  Selector : Selector  InputPortWidth=3  IndexOptions=Index vector (dialog)  Indices=[2]  OutputSizes=1
  Stop Simulation : Stop
  Terminator : Terminator
  Terminator1 : Terminator
  To Workspace1 : ToWorkspace  VariableName=SensorBodyFrame  SampleTime=-1
      settings: Save2DSignal=2-D array (concatenate along first dimension)
  To Workspace2 : ToWorkspace  VariableName=xyzHAT  SampleTime=-1
      settings: Save2DSignal=2-D array (concatenate along first dimension)
  "Trunk Sensor " : Subsystem
  frame : PMIOPort  Side=Left
  Right Hip : PMIOPort  Port=2  Side=Left
  Left Hip : PMIOPort  Port=3  Side=Left
  tag scope: AnklePosL_rot=global, AnklePosR_rot=global, CoM_Position=global, CoM_Velocity=global, CoM_Velocity_rot=global, HipL=global, HipR=global, R_body=global, RotationTrunk=global, RotationVelocityTrunk=global, TRK_CG=global, TrunkRotVel_lat=global, TrunkRotVel_sag=global, TrunkRot_lat=global, TrunkRot_sag=global
  wires:
  Selector/1 -> Compare To Constant/1
  Compare To Constant/1 -> Stop Simulation/1
  "Trunk Sensor "/2(Velocity Trunk [m/s]) -> Align Axis/5(Velocity Trunk [m/s]), [CoM_Velocity]
  "Trunk Sensor "/4(Rotation Trunk [rad]) -> [RotationTrunk]
  Ankle Position Right [m]/1 -> Align Axis/1(Ankle Position Right [m])
  "  XYZ Sensor Right Hip"/1(Hip Position [m]) -> [HipR], R Movement direction/1(Hip Right), Align Axis/7(Hip Position Right [m])
  R Movement direction/1("R ") -> [R_body], Align Axis/3("R ")
  Ankle Position Left [m]/1 -> Align Axis/2(Ankle Position Left [m])
  "Trunk Sensor "/1(Position Trunk [m]) -> [TRK_CG], Selector/1, To Workspace2/1, Align Axis/4(Position Trunk [m]), [CoM_Position]
  "  XYZ Sensor Left Hip"/1(Hip Position [m]) -> [HipL], Align Axis/6(Hip Position Left [m]), R Movement direction/2(Hip Left)
  "Trunk Sensor "/3(Rotation Velocity Trunk [rad/s]) -> [RotationVelocityTrunk]
  Mux/1 -> To Workspace1/1
  "  XYZ Sensor Right Hip"/2(Hip Velocity [m/s]) -> Terminator/1
  "  XYZ Sensor Left Hip"/2(Hip Velocity [m/s]) -> Terminator1/1
  Align Axis/1(Ankle Position Left (body frame)) -> [AnklePosL_rot], Mux/1
  Align Axis/2(Ankle Position Right (body frame)) -> [AnklePosR_rot], Mux/2
  Align Axis/3(Trunk Velocity (body frame)) -> [CoM_Velocity_rot], Mux/3
  Align Axis/4(Saggital Trunk Rotation [rad] (body frame)) -> [TrunkRot_sag], Mux/4
  Align Axis/5(Lateral Trunk Rotation [rad] (body frame)) -> [TrunkRot_lat], Mux/5
  Align Axis/6(Saggital Trunk Rotation Velocity [rad/s] (body frame)) -> [TrunkRotVel_sag], Mux/6
  Align Axis/7(Lateral Trunk Rotation Velocity [rad/s] (body frame)) -> [TrunkRotVel_lat], Mux/7
  connections:
  "Trunk Sensor "/LConn1 -- frame/RConn1
  "  XYZ Sensor Left Hip"/LConn1 -- Left Hip/RConn1
  "  XYZ Sensor Right Hip"/LConn1 -- Right Hip/RConn1

== system nms3D_2021/Body and Contact Model/World Frame ==
  Mechanism Configuration : sm_lib/Utilities/Mechanism Configuration  UniformGravity=Constant  GravityVector=[0 -9.81 0]  GravityVectorUnits=m/s^2  GravityUnits=m/s^2  LinearizationDelta=0.001  JointModeTransitionNonlinearIterations=2
  Solver Configuration : nesl_utility/Solver Configuration  PhysicalDomain=network_engine_domain  SubClassName=solver  LeftPortType=input  RightPortType=generic  Tones=[]  Harmonics=[]  SimulateNoise=off  Profile=off  UseLocalSampling=off  EnableSwitchedLinearOptims=on  FrequencyDomain=off  UseCCode=off  RelTol=0.001  AbsTol=1e-06  MinStep=1e-09  ToWorkspace=off  RevertToSquareIcSolve=off  NumHomotopyIterations=100  PhasorMode=off  PhasorModeNumHarmonics=1  DoDC=off  ResidualTolerance=1e-9  UseLocalSolver=off  LocalSolverChoice=NE_BACKWARD_EULER_ADVANCER  LocalSolverSampleTime=.001  DoFixedCost=off  MaxNonlinIter=3  MaxModeIter=2  ComputeImpulses=off  ImpulseIterations=2  LinearAlgebra=Sparse  EquationFormulation=NE_TIME_EF  DelaysMemoryBudget=1024  AutomaticFiltering=on  FilteringTimeConstant=0.001  PartitionStorageMethod=AS_NEEDED  PartitionMemoryBudget=1024  PartitionMethod=FAST
      settings: SourceProductBaseCode=PW,SS
  World Frame : sm_lib/Frames and Transforms/World Frame
  Conn1 : PMIOPort  Side=Right
  connections:
  Solver Configuration/RConn1 -- Mechanism Configuration/RConn1 -- Conn1/RConn1 -- World Frame/RConn1

== system nms3D_2021/CMA Data/SS_dist1 ==
  In1 : Inport
  Trigger : TriggerPort  VariantControl=(inherit)  ZeroCross=off
  To Current Workspace4 : ToWorkspace  VariableName=SSdist  SaveFormat=Structure With Time  SampleTime=-1
      settings: MaxDataPoints=3
  wires:
  In1/1 -> To Current Workspace4/1

== system nms3D_2021/CMA Data/Step Counter ==
  Step2 : Inport
  Step1 : Inport  Port=2
  Constant1 : Constant  Value=0
  Constant2 : Constant  Value=0
  Constant3 : Constant  Value=0
  Constant4 : Constant  Value=-1
  Saturation Dynamic : simulink/Discontinuities/Saturation Dynamic  OutMin=[]  OutMax=[]  OutDataTypeStr=Inherit: Same as second input  OutDataType=fixdt(1, 16)  OutScaling=2^-10  DoSatur=off
  Saturation Dynamic1 : simulink/Discontinuities/Saturation Dynamic  OutMin=[]  OutMax=[]  OutDataTypeStr=Inherit: Same as second input  OutDataType=fixdt(1, 16)  OutScaling=2^-10  DoSatur=off
  Sum : Sum  Inputs=|++
  Sum1 : Sum  Inputs=++|
  Sum2 : Sum  Inputs=|++
  count steps1 : Subsystem  TreatAsAtomicUnit=on
  count steps2 : Subsystem  TreatAsAtomicUnit=on
  nStep : Outport  VectorParamsAs1DForOutWhenUnconnected=off
  wires:
  count steps1/1(nStep) -> Saturation Dynamic1/2, Sum2/2, Sum/2
  count steps2/1(nStep) -> Saturation Dynamic/2, Sum1/1, Sum/1
  Constant3/1 -> Saturation Dynamic/3
  Saturation Dynamic/1 -> count steps2/1(nStep-1)
  Constant1/1 -> Sum1/2
  Sum1/1 -> Saturation Dynamic1/1
  Constant2/1 -> Saturation Dynamic1/3
  Saturation Dynamic1/1 -> count steps1/1(nStep-1)
  Constant4/1 -> Sum2/1
  Sum2/1 -> Saturation Dynamic/1
  Step2/1 -> count steps2/Trigger
  Sum/1 -> nStep/1
  Step1/1 -> count steps1/Trigger

== system nms3D_2021/CMA Data/check steady state ==
  p : Inport
  nStep : Inport  Port=2
  Abs : Abs  ZeroCross=off
  Add{,1..9,15..16} (12 alike) : Sum  Inputs=-+
  Add{10..14,17} (6 alike) : Sum  Inputs=+-
  Demux2 : Demux  Outputs=7
  Demux3 : Demux  Outputs=7
  Fcn : Fcn  Expr=rem(u(1), 2)
  Gain14 : Gain  Gain=.5
  Mux1 : Mux  Inputs=6
  Rounding Function1 : Rounding
  Sum of Elements : Sum  Inputs=+
  even : Subsystem  TreatAsAtomicUnit=on
  odd : Subsystem  TreatAsAtomicUnit=on
  SS_dist : Outport  VectorParamsAs1DForOutWhenUnconnected=off
  wires:
  p/1 -> even/1(In1), odd/1(In1)
  Fcn/1 -> odd/Trigger, even/Trigger
  odd/1(Out1) -> Demux2/1
  even/1(Out1) -> Demux3/1
  Add10/1 -> Mux1/1
  Add11/1 -> Mux1/2
  Add12/1 -> Mux1/3
  Add13/1 -> Mux1/4
  Add14/1 -> Mux1/5
  Demux2/2 -> Add/2
  Demux2/3 -> Add1/2
  Demux2/4 -> Add2/2
  Demux2/5 -> Add3/2
  Demux2/6 -> Add4/2
  Demux2/1 -> Add/1, Add1/1, Add2/1, Add3/1, Add4/1, Add15/1
  Demux3/2 -> Add5/2
  Demux3/3 -> Add6/2
  Demux3/4 -> Add7/2
  Demux3/5 -> Add8/2
  Demux3/6 -> Add9/2
  Demux3/1 -> Add5/1, Add6/1, Add7/1, Add8/1, Add9/1, Add16/1
  Add/1 -> Add10/1
  Add1/1 -> Add11/1
  Add2/1 -> Add12/1
  Add3/1 -> Add13/1
  Add4/1 -> Add14/1
  Add5/1 -> Add10/2
  Add6/1 -> Add11/2
  Add7/1 -> Add12/2
  Add8/1 -> Add13/2
  Add9/1 -> Add14/2
  Mux1/1 -> Abs/1
  Abs/1 -> Sum of Elements/1
  Sum of Elements/1 -> SS_dist/1
  nStep/1 -> Gain14/1
  Gain14/1 -> Rounding Function1/1
  Rounding Function1/1 -> Fcn/1
  Demux2/7 -> Add15/2
  Demux3/7 -> Add16/2
  Add15/1 -> Add17/1
  Add16/1 -> Add17/2
  Add17/1 -> Mux1/6

== system nms3D_2021/Muscle Actuation Layer/Muscles Left ==
  STIM Left : Inport
  Demux : Demux  Outputs=5
  Muscle Dynamics (Vectorized)1 : Subsystem
  Muscle Length Vector1 : Subsystem
  Muscle Torque Contributions1 : Subsystem
  Scope : Scope
  Scope1 : Scope
  Terminator : Terminator
  Terminator1 : Terminator
  tauHipPitchL : Outport
  tauHipRollL : Outport  Port=2
  tauKneeL : Outport  Port=3
  tauAnkleRollL : Outport  Port=4
  tauAnklePitchL : Outport  Port=5
  "Leg Torque " : Outport  Port=6
  tag scope: LFmVec=global, LLceVec=global, LVceVec=global
  wires:
  Demux/2 -> Muscle Length Vector1/2(qHipRoll [rad])
  Muscle Torque Contributions1/2(tauHR [Nm]) -> tauHipRollL/1
  Demux/1 -> Muscle Length Vector1/1(qHipPitch [rad])
  Demux/4 -> Muscle Length Vector1/4(qAnkleRoll [rad])  "qA"
  Muscle Dynamics (Vectorized)1/3(Vce) -> [LVceVec]
  Muscle Torque Contributions1/3(tauK [Nm]) -> tauKneeL/1
  Demux/3 -> Muscle Torque Contributions1/1(qKnee [rad]), Muscle Length Vector1/3(qKnee [rad])  "qK"
  Muscle Dynamics (Vectorized)1/5(ForceLengthFactor) -> Terminator1/1
  Muscle Length Vector1/1(lmtc [m x11]) -> Muscle Dynamics (Vectorized)1/1(lmtc [m])
  Muscle Torque Contributions1/1(tauHP [Nm]) -> tauHipPitchL/1
  Muscle Torque Contributions1/5(tauA [Nm]) -> tauAnklePitchL/1
  Muscle Dynamics (Vectorized)1/4(A) -> Terminator/1
  Muscle Dynamics (Vectorized)1/2(Lce) -> [LLceVec]
  STIM Left/1 -> Scope/1, Muscle Dynamics (Vectorized)1/2(STIM)
  [Llegq] -> Demux/1
  Muscle Torque Contributions1/6(Leg Torque) -> "Leg Torque "/1
  Muscle Dynamics (Vectorized)1/1(Fmtc) -> Scope1/1, Muscle Torque Contributions1/3(FmVec [N x11]), [LFmVec]
  Demux/5 -> Muscle Torque Contributions1/2(qAnkle [rad]), Muscle Length Vector1/5(qAnkle Pitch [rad])
  Muscle Torque Contributions1/4(tauAR [Nm]) -> tauAnkleRollL/1

== system nms3D_2021/Muscle Actuation Layer/Muscles Right ==
  STIM Right : Inport
  Demux : Demux  Outputs=5
  Goto15 : Goto  Commented=on  GotoTag=activation_R  TagVisibility=global
  Muscle Dynamics (Vectorized) : Subsystem
  Muscle Length Vector : Subsystem  Commented=on
  Muscle Length Vector Right : Subsystem
  Muscle Torque Contributions : Subsystem
  R Leg Muscles Vce [m/s x11]1 : Goto  Commented=on  GotoTag=RForceLength  TagVisibility=global
  Scope : Scope
  Scope1 : Scope
  tauHipPitchR : Outport
  tauHipRollR : Outport  Port=2
  tauKneeR : Outport  Port=3
  tauHipAnkleRollR : Outport  Port=4
  tauHipAnklePitchR : Outport  Port=5
  Leg Torque : Outport  Port=6
  tag scope: RFmVec=global, RLceVec=global, RVceVec=global
  wires:
  Muscle Torque Contributions/3(tauK [Nm]) -> tauKneeR/1
  Muscle Length Vector Right/1(lmtc [m x11]) -> Muscle Dynamics (Vectorized)/1(lmtc [m])
  Demux/3 -> Muscle Length Vector Right/3(qKnee [rad]), Muscle Torque Contributions/1(qKnee [rad])  "qK"
  Muscle Dynamics (Vectorized)/2(Lce) -> [RLceVec]
  Muscle Torque Contributions/2(tauHR [Nm]) -> tauHipRollR/1
  Demux/1 -> Muscle Length Vector Right/1(qHipPitch [rad])  "qHP"
  Muscle Dynamics (Vectorized)/5(ForceLengthFactor) -> R Leg Muscles Vce [m/s x11]1/1
  Muscle Dynamics (Vectorized)/1(Fmtc) -> Scope/1, Muscle Torque Contributions/3(FmVec [N x11]), [RFmVec]
  Muscle Dynamics (Vectorized)/4(A) -> Goto15/1
  Muscle Dynamics (Vectorized)/3(Vce) -> [RVceVec]
  Muscle Torque Contributions/1(tauHP [Nm]) -> tauHipPitchR/1
  Demux/2 -> Muscle Length Vector Right/2(qHipRoll [rad])  "qHR"
  STIM Right/1 -> Scope1/1, Muscle Dynamics (Vectorized)/2(STIM)
  [Rlegq] -> Demux/1  "qHP"
  Muscle Torque Contributions/6(Leg Torque) -> Leg Torque/1
  Demux/5 -> Muscle Length Vector Right/5(qAnkle Pitch [rad]), Muscle Torque Contributions/2(qAnkle [rad])
  Demux/4 -> Muscle Length Vector Right/4(qAnkleRoll [rad])  "qA"
  Muscle Torque Contributions/4(tauAR [Nm]) -> tauHipAnkleRollR/1
  Muscle Torque Contributions/5(tauA [Nm]) -> tauHipAnklePitchR/1
